simulink model "inverter"  (R2022b)
settings: Solver=VariableStepAuto  StartTime=0.0  StopTime=1  RelTol=1e-3
libraries: spsMosfetLib x4, spsVoltageMeasurementLib x2, spsDCVoltageSourceLib x1, spsSeriesRLCBranchLib x1, sps_lib x1
settings Model: Creator=Shantanu  LastModifiedBy=Shantanu

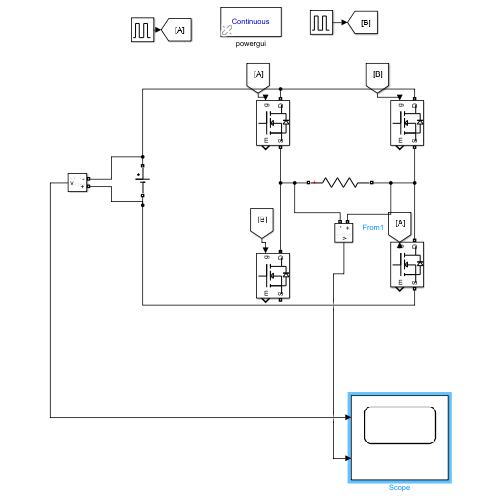
[thumbnail: Simulink's stored preview of the top-level diagram]
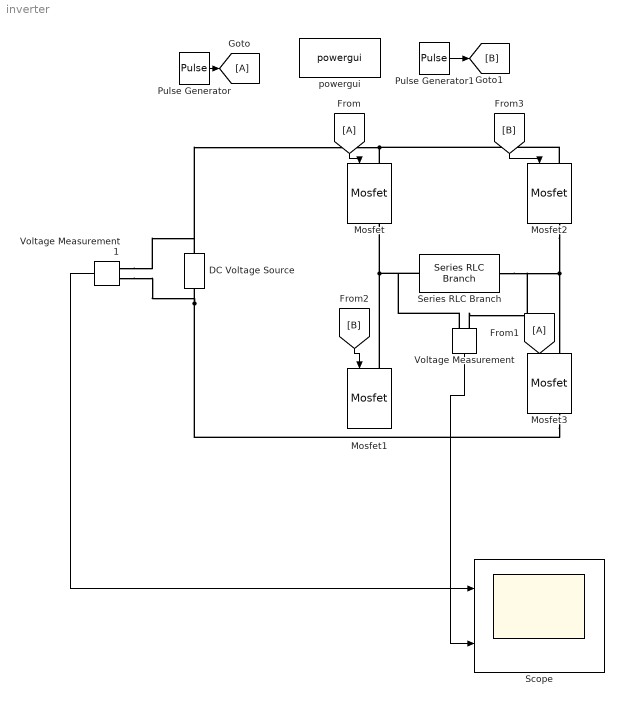
== system inverter ==
  DC Voltage Source : spsDCVoltageSourceLib/DC Voltage Source  Amplitude=200  Measurements=None
  From : From
  From1 : From
  Goto : Goto
  Mosfet{,1..3} (4 alike) : spsMosfetLib/Mosfet  Ron=0.1  Lon=0  Rd=0.01  Vfd=0  IC=0  Rs=1e5  Cs=inf  Measurements=on
  Pulse Generator : DiscretePulseGenerator  PulseType=Time based  Period=2e-3  PulseWidth=50
  Pulse Generator1 : DiscretePulseGenerator  PulseType=Time based  Period=2e-3  PulseWidth=50  PhaseDelay=1e-3
  Scope : Scope  NumInputPorts=2
  Series RLC Branch : spsSeriesRLCBranchLib/Series RLC Branch  LConnTagsString=__new0  RConnTagsString=__new0  BranchType=R  Resistance=50  Inductance=1e-3  SetiL0=off  InitialCurrent=0  Capacitance=1e-6  Setx0=off  InitialVoltage=0  Measurements=None
  Voltage Measurement : spsVoltageMeasurementLib/Voltage Measurement  PhasorSimulation=off  OutputType=Complex  PSBequivalent=0
  Voltage Measurement1 : spsVoltageMeasurementLib/Voltage Measurement  PhasorSimulation=off  OutputType=Complex  PSBequivalent=0
  powergui : sps_lib/powergui  Priority=1  SimulationMode=Continuous  SampleTime=50e-6  frequency=60  Iterations=50  frequencyindice=0  Pbase=100e6  ErrMax=1e-4  UnitsV=kV  UnitsW=MW  buscounter=0  FunctionMessages=off  echomessages=off  EnableUseOfTLC=off  CurrentSourceSwitches=off  DisableSnubberDevices=off  DisableRonSwitches=off  DisableVfSwitches=off  DisplayEquations=off  AutomaticDiscreteSolvers=off  SolverType=Tustin/Backward Euler (TBE)  Interpol=off  ExternalGateDelay=off  methode=off  Ts=100  x0status=blocks  SPID=on  SwTol=0  HookPort=off  NonlinearTolerance=1e-4  nMaxIteration=100  ContinueOnMaxIteration=off  RestoreLinks=warning  ResistiveCurrentMeasurement=off  Frange=[0:2:500]  Ylog=off  Xlog=on  ShowGrid=off  save=off  variable=ZData  structure=0  ZoomFFT=off  StartTime=0.0  cycles=1  DisplayStyle=1  fundamental=60  FreqAxis=off  MaxFrequency=1000  frequencyindicesteady=1  RmsSteady=1  display=off
  wires:
  Pulse Generator/1 -> Goto/1
  From/1 -> Mosfet/1
  From1/1 -> Mosfet3/1
  Pulse Generator1/1 -> [B]
  [B] -> Mosfet1/1
  [B] -> Mosfet2/1
  Voltage Measurement1/1 -> Scope/1
  Voltage Measurement/1 -> Scope/2
  connections:
  Mosfet3/RConn1 -- Voltage Measurement1/LConn1 -- DC Voltage Source/LConn1
  Mosfet1/LConn1 -- Voltage Measurement/LConn2 -- Series RLC Branch/LConn1 -- Mosfet/RConn1
  Mosfet2/RConn1 -- Voltage Measurement/LConn1 -- Series RLC Branch/RConn1 -- Mosfet3/LConn1
  Mosfet/LConn1 -- Voltage Measurement1/LConn2 -- DC Voltage Source/RConn1 -- Mosfet2/LConn1
